simulink model "mcb_pmsm_foc_f28379d_dyno"  (R2024b)
settings: Solver=FixedStepDiscrete  StartTime=0.0  StopTime=10  RelTol=1e-3  EnableMultiTasking=on
InitFcn:
  | mcb_pmsm_foc_dyno_f28379d_data;
model workspace (MAT data in the model file):
  encoderResolution = 2000
  hallOffset = '0.5'
  indexOffset = 850
  polePairs = '4'
values from neighbouring files (symbols this model uses):
  dataType = 'single'    [mcb_pmsm_foc_dyno_f28379d_data.m]
  inverter_motor1 = mcb_updateInverterParameters(pmsm_motor1,inverter_motor1,target)    [mcb_pmsm_foc_dyno_f28379d_data.m]
  inverter_motor2 = mcb_updateInverterParameters(pmsm_motor2,inverter_motor2,target)    [mcb_pmsm_foc_dyno_f28379d_data.m]
  PI_params_motor1 = calculate_PI_params(pmsm_motor1,inverter_motor1)    [mcb_pmsm_foc_dyno_f28379d_data.m]
  PI_params_motor2 = calculate_PI_params(pmsm_motor2,inverter_motor2)    [mcb_pmsm_foc_dyno_f28379d_data.m]
  pmsm_motor1 = mcb_SetPMSMMotorParameters('Teknic2310P')    [mcb_pmsm_foc_dyno_f28379d_data.m]
  pmsm_motor2 = mcb_SetPMSMMotorParameters('Teknic2310P')    [mcb_pmsm_foc_dyno_f28379d_data.m]
  PU_System_motor1 = mcb_SetPUSystem(pmsm_motor1,inverter_motor1)    [mcb_pmsm_foc_dyno_f28379d_data.m]
  PU_System_motor2 = mcb_SetPUSystem(pmsm_motor2,inverter_motor2)    [mcb_pmsm_foc_dyno_f28379d_data.m]
  T_pwm = 1/PWM_frequency    (= 5e-05)    [mcb_pmsm_foc_dyno_f28379d_data.m]
  target = mcb_SetProcessorDetails('F28379D',PWM_frequency)    [mcb_pmsm_foc_dyno_f28379d_data.m]
  Ts = T_pwm    (= 5e-05)    [mcb_pmsm_foc_dyno_f28379d_data.m]
  Ts_inverter = T_pwm/2    (= 2.5e-05)    [mcb_pmsm_foc_dyno_f28379d_data.m]
  Ts_motor = T_pwm/2    (= 2.5e-05)    [mcb_pmsm_foc_dyno_f28379d_data.m]
  Ts_speed = 10*Ts    (= 0.0005)    [mcb_pmsm_foc_dyno_f28379d_data.m]
undefined symbols (not defined in the file or in its folder): DiscIntNeverNeededParam, Down, GPTRIP1SEL, GPTRIP2SEL, TZ1, TZ2, Up
libraries: mcbcontrolslib x22, c2802xlib x14, simulink x10, c2837xDlib x7, mcbpositiondecoderlib x6, slpidlib x5, c280xlib x5, mcbpmsmnonlinearlib x4, svdschedulerlib x3, autolibpmsmexterior x2, mcbplantlib x2, svdutilitieslib x1
(part 4 of 4)

== system mcb_pmsm_foc_f28379d_dyno/Current control for motor1/Control_System/Closed Loop Control/Current_Controllers/PI_Controller_Iq ==
  I_ref : Inport
  I_fb : Inport  Port=2
  Constant : Constant
  Data Store Read1 : DataStoreRead  DataStoreName=EnMtrCtrl  IndexOptions=Index vector (dialog)  Indices=1  OutputSizes=1
  Discrete PI Controller with anti-windup & reset : slpidlib/PID Controller  Controller=PI  Form=Parallel  TimeDomain=Discrete-time  UseExternalTs=off  SampleTime=-1  IntegratorMethod=Forward Euler  FilterMethod=Forward Euler  ControllerParametersSource=external  P=1  I=1  UseKiTs=on  D=0  UseExternalDerivativeSource=off  N=100  UseFilter=on  TunerSelectOption=Transfer Function Based (PID Tuner App)  InitialConditionSource=external  InitialConditionForIntegrator=0  InitialConditionForFilter=0  DifferentiatorICPrevScaledInput=0  ExternalReset=level  TrackingMode=off  Kt=1  LimitOutput=on  SatLimitsSource=internal  UpperSaturationLimit=1  LowerSaturationLimit=-1  LinearizeAsGain=on  AntiWindupMode=clamping  Kb=1  LimitIntegrator=off  UpperIntegratorSaturationLimit=inf  LowerIntegratorSaturationLimit=-inf  RndMeth=Simplest  POutMin=[]  POutMax=[]  IOutMin=[]  IOutMax=[]  DOutMin=[]  DOutMax=[]  NOutMin=[]  NOutMax=[]  SumOutMin=[]  SumOutMax=[]  SaturationOutDataTypeStr=Inherit: Inherit via back propagation  SaturationOutMin=[]  SaturationOutMax=[]  PParamMin=[]  PParamMax=[]  IParamMin=[]  IParamMax=[]  DParamMin=[]  DParamMax=[]  NParamMin=[]  NParamMax=[]  KbParamMin=[]  KbParamMax=[]  KtParamMin=[]  KtParamMax=[]  KbOutMin=[]  KbOutMax=[]  KtOutMin=[]  KtOutMax=[]  IntegratorOutMin=[]  IntegratorOutMax=[]  FilterOutMin=[]  FilterOutMax=[]  SumI1OutMin=[]  SumI1OutMax=[]  SumI2OutMin=[]  SumI2OutMax=[]  SumI3OutMin=[]  SumI3OutMax=[]  SumI4OutMin=[]  SumI4OutMax=[]  SumDOutMin=[]  SumDOutMax=[]  DifferentiatorOutMin=[]  DifferentiatorOutMax=[]  FilterDiffOutCoefMin=[]  FilterDiffOutCoefMax=[]  ReciprocalOutMin=[]  ReciprocalOutMax=[]  SumDenOutMin=[]  SumDenOutMax=[]  SumNumOutMin=[]  SumNumOutMax=[]  DivideOutMin=[]  DivideOutMax=[]  UdiffTsProdOutMin=[]  UdiffTsProdOutMax=[]  NTsProdOutMin=[]  NTsProdOutMax=[]  UintegralTsProdOutMin=[]  UintegralTsProdOutMax=[]  UngainTsProdOutMin=[]  UngainTsProdOutMax=[]  ClampingZeroOutDataTypeStr=Inherit: Inherit via back propagation  ClampingZeroOutMin=[]  ClampingZeroOutMax=[]  FilterDenConstantOutDataTypeStr=Inherit: Inherit via back propagation  FilterDenConstantOutMin=[]  FilterDenConstantOutMax=[]  PCopyOutDataTypeStr=Inherit: Inherit via back propagation  PCopyOutMin=[]  PCopyOutMax=[]  NCopyOutDataTypeStr=Inherit: Inherit via back propagation  NCopyOutMin=[]  NCopyOutMax=[]  IntegratorContinuousStateAttributes=''  IntegratorStateMustResolveToSignalObject=off  IntegratorRTWStateStorageClass=Auto  FilterContinuousStateAttributes=''  FilterStateMustResolveToSignalObject=off  FilterRTWStateStorageClass=Auto  ParallelPVariant=ExternalParameters  IdealPVariant=Disabled  IVariant=ExternalParameters  DVariant=Disabled  IntegratorVariant=Discrete  SatVariant=Enabled  AWVariant=DiscClampingParallel  PCopyVariant=Disabled  TRVariant=Disabled  FdbkBlocksVariant=Forward  IdealPFdbkVariant=Disabled  SatFdbkVariant=Disabled  DerivativeFilterVariant=Disabled  NVariant=Disabled  NCopyVariant=Disabled_SignalSpec  FilterICVariant=Disabled  IntegratorICVariant=ExternalICs  ExternalResetVariant=ExternalReset  TRSumVariant=Passthrough  SumFdbkVariant=Disabled  SumVariant=Sum_PI  TsampFilterVariant=InternalTs  TsampNgainVariant=Passthrough  TsampIntegralVariant=Disabled_SignalSpec  ExternalSaturationOutDataTypeStr=Inherit: Same as second input  DerivativeSourceVariant=Disabled  PreIntVariant=InternalPreInt
  Ki : Constant  Value=PI_params_motor1.Ki_i*Ts  OutDataTypeStr=dataType  SampleTime=-1
  Kp : Constant  Value=PI_params_motor1.Kp_i  OutDataTypeStr=dataType  SampleTime=-1
  Kp1 : Constant  Value=0  OutDataTypeStr=dataType  SampleTime=-1
  Logical Operator : Logic  Operator=NOT  IconShape=distinctive  AllPortsSameDT=off  OutDataTypeStr=boolean
  MATLAB Function : MATLAB Function  TreatAsAtomicUnit=on
  Sum : Sum  Inputs=|+-  OutDataTypeStr=Inherit: Same as first input
  V_ref : Outport  VectorParamsAs1DForOutWhenUnconnected=off
  wires:
  MATLAB Function/1(V_q_ref) -> V_ref/1
  Data Store Read1/1 -> Logical Operator/1
  I_fb/1 -> Sum/2
  I_ref/1 -> Sum/1
  Kp/1 -> MATLAB Function/2(P)
  Sum/1 -> MATLAB Function/1(e)
  Ki/1 -> MATLAB Function/3(I_Ts_speed)
  Logical Operator/1 -> MATLAB Function/4(reset)
  Kp1/1 -> MATLAB Function/5(Iq0)
  Constant/1 -> MATLAB Function/6(saturation_limit)

== system mcb_pmsm_foc_f28379d_dyno/Current control for motor1/Input Scaling/Calculate Phase Currents/Data_Type/Data_Type_Fixed_Point ==
  In1 : Inport
  Data Type Conversion : DataTypeConversion  OutDataTypeStr=fixdt(1,32,17)  ConvertRealWorld=Stored Integer (SI)  RndMeth=Simplest  SaturateOnIntegerOverflow=off
  Data Type Conversion1 : DataTypeConversion  OutDataTypeStr=dataType  RndMeth=Simplest  SaturateOnIntegerOverflow=off
  Q17 per unit conversion : ArithShift  BitShiftNumber=-6
  Iab_meas_PU : Outport
  wires:
  In1/1 -> Q17 per unit conversion/1
  Data Type Conversion1/1 -> Iab_meas_PU/1
  Data Type Conversion/1 -> Data Type Conversion1/1
  Q17 per unit conversion/1 -> Data Type Conversion/1

== system mcb_pmsm_foc_f28379d_dyno/Current control for motor1/Input Scaling/Calculate Phase Currents/Data_Type/Data_Type_Float ==
  In1 : Inport
  Get ADC Voltage : Gain  Gain=target.ADC_Vref /target.ADC_MaxCount  OutDataTypeStr=dataType  RndMeth=Simplest
  Get Currents : Gain  Gain=1/inverter_motor1.ISenseVoltPerAmp  RndMeth=Simplest  OutDataTypeStr=Inherit: Same as input
  PU_Conversion : Gain  Gain=1/PU_System_motor1.I_base  RndMeth=Simplest  OutDataTypeStr=Inherit: Same as input
  Iab_meas_PU : Outport
  wires:
  Get ADC Voltage/1 -> Get Currents/1
  Get Currents/1 -> PU_Conversion/1
  PU_Conversion/1 -> Iab_meas_PU/1
  In1/1 -> Get ADC Voltage/1

== system mcb_pmsm_foc_f28379d_dyno/Current control for motor1/SCI_Tx/Code Generation/Data_Conditioning_Tx/Data_Type_Fixed_Point ==
  In1 : Inport
  Data Type Conversion : DataTypeConversion  OutDataTypeStr=fixdt(1,32,28)  RndMeth=Simplest  SaturateOnIntegerOverflow=off
  Data Type Conversion3 : DataTypeConversion  OutDataTypeStr=uint32  ConvertRealWorld=Stored Integer (SI)  RndMeth=Simplest  SaturateOnIntegerOverflow=off
  Data_Log : Outport
  wires:
  In1/1 -> Data Type Conversion/1
  Data Type Conversion3/1 -> Data_Log/1
  Data Type Conversion/1 -> Data Type Conversion3/1

== system mcb_pmsm_foc_f28379d_dyno/Current control for motor1/SCI_Tx/Code Generation/Data_Conditioning_Tx/Data_Type_Float ==
  In1 : Inport
  Byte Pack : svdutilitieslib/Byte Pack  maskPackedDataType=uint32  datatypes={'single'}  byteAlign=4  blockPlatform=tic2000
  Data_Log : Outport
  wires:
  Byte Pack/1 -> Data_Log/1
  In1/1 -> Byte Pack/1

== system mcb_pmsm_foc_f28379d_dyno/Current control for motor1/SCI_Tx/Code Generation/Data_Logging/Data ==
  Data : Inport
  Data_width : Inport  Port=2
  Action Port : ActionPort  ActionPortLabel=else
  Dummy : Constant  Value=hex2dec('0000')  OutDataTypeStr=uint32
  Mux : Mux  Inputs=2
  Data_out : Outport  VectorParamsAs1DForOutWhenUnconnected=off
  Iteration : Outport  Port=2  VectorParamsAs1DForOutWhenUnconnected=off
  wires:
  Data_width/1 -> Iteration/1
  Data/1 -> Mux/1
  Dummy/1 -> Mux/2
  Mux/1 -> Data_out/1

== system mcb_pmsm_foc_f28379d_dyno/Current control for motor1/SCI_Tx/Code Generation/Data_Logging/End ==
  Data : Inport
  Data_width : Inport  Port=2
  Action Port : ActionPort  ActionPortLabel=elseif(u1 == 599)
  Bias : Bias  Bias=1  SaturateOnIntegerOverflow=off
  End : Constant  Value=hex2dec('45454545')  OutDataTypeStr=uint32
  Mux : Mux  Inputs=2
  Data_out : Outport  VectorParamsAs1DForOutWhenUnconnected=off
  Iteration : Outport  Port=2  VectorParamsAs1DForOutWhenUnconnected=off
  wires:
  Data/1 -> Mux/1
  Data_width/1 -> Bias/1
  Bias/1 -> Iteration/1
  End/1 -> Mux/2
  Mux/1 -> Data_out/1

== system mcb_pmsm_foc_f28379d_dyno/Current control for motor1/SCI_Tx/Code Generation/Data_Logging/Start ==
  Data : Inport
  Data_width : Inport  Port=2
  Action Port : ActionPort  ActionPortLabel=if(u1 == 0)
  Bias : Bias  Bias=1  SaturateOnIntegerOverflow=off
  Mux : Mux  Inputs=2
  Start : Constant  Value=hex2dec('53535353')  OutDataTypeStr=uint32
  Data_out : Outport  VectorParamsAs1DForOutWhenUnconnected=off
  Iteration : Outport  Port=2  VectorParamsAs1DForOutWhenUnconnected=off
  wires:
  Data/1 -> Mux/2
  Data_width/1 -> Bias/1
  Bias/1 -> Iteration/1
  Start/1 -> Mux/1
  Mux/1 -> Data_out/1

== system mcb_pmsm_foc_f28379d_dyno/Current control for motor2/Control_System/Closed Loop Control/Current_Controllers/PI_Controller_Id ==
  I_ref : Inport
  I_fb : Inport  Port=2
  Constant : Constant
  Data Store Read1 : DataStoreRead  DataStoreName=EnMtr2TrqCtrl  IndexOptions=Index vector (dialog)  Indices=1  OutputSizes=1
  Discrete PI Controller with anti-windup & reset : slpidlib/PID Controller  Controller=PI  Form=Parallel  TimeDomain=Discrete-time  UseExternalTs=off  SampleTime=-1  IntegratorMethod=Forward Euler  FilterMethod=Forward Euler  ControllerParametersSource=external  P=1  I=1  UseKiTs=on  D=0  UseExternalDerivativeSource=off  N=100  UseFilter=on  TunerSelectOption=Transfer Function Based (PID Tuner App)  InitialConditionSource=external  InitialConditionForIntegrator=0  InitialConditionForFilter=0  DifferentiatorICPrevScaledInput=0  ExternalReset=level  TrackingMode=off  Kt=1  LimitOutput=on  SatLimitsSource=internal  UpperSaturationLimit=1  LowerSaturationLimit=-1  LinearizeAsGain=on  AntiWindupMode=clamping  Kb=1  LimitIntegrator=off  UpperIntegratorSaturationLimit=inf  LowerIntegratorSaturationLimit=-inf  RndMeth=Simplest  POutMin=[]  POutMax=[]  IOutMin=[]  IOutMax=[]  DOutMin=[]  DOutMax=[]  NOutMin=[]  NOutMax=[]  SumOutMin=[]  SumOutMax=[]  SaturationOutDataTypeStr=Inherit: Inherit via back propagation  SaturationOutMin=[]  SaturationOutMax=[]  PParamMin=[]  PParamMax=[]  IParamMin=[]  IParamMax=[]  DParamMin=[]  DParamMax=[]  NParamMin=[]  NParamMax=[]  KbParamMin=[]  KbParamMax=[]  KtParamMin=[]  KtParamMax=[]  KbOutMin=[]  KbOutMax=[]  KtOutMin=[]  KtOutMax=[]  IntegratorOutMin=[]  IntegratorOutMax=[]  FilterOutMin=[]  FilterOutMax=[]  SumI1OutMin=[]  SumI1OutMax=[]  SumI2OutMin=[]  SumI2OutMax=[]  SumI3OutMin=[]  SumI3OutMax=[]  SumI4OutMin=[]  SumI4OutMax=[]  SumDOutMin=[]  SumDOutMax=[]  DifferentiatorOutMin=[]  DifferentiatorOutMax=[]  FilterDiffOutCoefMin=[]  FilterDiffOutCoefMax=[]  ReciprocalOutMin=[]  ReciprocalOutMax=[]  SumDenOutMin=[]  SumDenOutMax=[]  SumNumOutMin=[]  SumNumOutMax=[]  DivideOutMin=[]  DivideOutMax=[]  UdiffTsProdOutMin=[]  UdiffTsProdOutMax=[]  NTsProdOutMin=[]  NTsProdOutMax=[]  UintegralTsProdOutMin=[]  UintegralTsProdOutMax=[]  UngainTsProdOutMin=[]  UngainTsProdOutMax=[]  ClampingZeroOutDataTypeStr=Inherit: Inherit via back propagation  ClampingZeroOutMin=[]  ClampingZeroOutMax=[]  FilterDenConstantOutDataTypeStr=Inherit: Inherit via back propagation  FilterDenConstantOutMin=[]  FilterDenConstantOutMax=[]  PCopyOutDataTypeStr=Inherit: Inherit via back propagation  PCopyOutMin=[]  PCopyOutMax=[]  NCopyOutDataTypeStr=Inherit: Inherit via back propagation  NCopyOutMin=[]  NCopyOutMax=[]  IntegratorContinuousStateAttributes=''  IntegratorStateMustResolveToSignalObject=off  IntegratorRTWStateStorageClass=Auto  FilterContinuousStateAttributes=''  FilterStateMustResolveToSignalObject=off  FilterRTWStateStorageClass=Auto  ParallelPVariant=ExternalParameters  IdealPVariant=Disabled  IVariant=ExternalParameters  DVariant=Disabled  IntegratorVariant=Discrete  SatVariant=Enabled  AWVariant=DiscClampingParallel  PCopyVariant=Disabled  TRVariant=Disabled  FdbkBlocksVariant=Forward  IdealPFdbkVariant=Disabled  SatFdbkVariant=Disabled  DerivativeFilterVariant=Disabled  NVariant=Disabled  NCopyVariant=Disabled_SignalSpec  FilterICVariant=Disabled  IntegratorICVariant=ExternalICs  ExternalResetVariant=ExternalReset  TRSumVariant=Passthrough  SumFdbkVariant=Disabled  SumVariant=Sum_PI  TsampFilterVariant=InternalTs  TsampNgainVariant=Passthrough  TsampIntegralVariant=Disabled_SignalSpec  ExternalSaturationOutDataTypeStr=Inherit: Same as second input  DerivativeSourceVariant=Disabled  PreIntVariant=InternalPreInt
  Ki : Constant  Value=PI_params_motor2.Ki_i*Ts  OutDataTypeStr=dataType  SampleTime=-1
  Ki1 : Constant  Value=0  OutDataTypeStr=dataType  SampleTime=-1
  Kp : Constant  Value=PI_params_motor2.Kp_i  OutDataTypeStr=dataType  SampleTime=-1
  Logical Operator : Logic  Operator=NOT  IconShape=distinctive  AllPortsSameDT=off  OutDataTypeStr=boolean
  MATLAB Function : MATLAB Function  TreatAsAtomicUnit=on
  Sum : Sum  Inputs=|+-  OutDataTypeStr=Inherit: Same as first input
  V_ref : Outport  VectorParamsAs1DForOutWhenUnconnected=off
  wires:
  Ki1/1 -> MATLAB Function/5(Id0)
  Logical Operator/1 -> MATLAB Function/4(reset)
  Ki/1 -> MATLAB Function/3(I_Ts_speed)
  Kp/1 -> MATLAB Function/2(P)
  Sum/1 -> MATLAB Function/1(e)
  MATLAB Function/1(V_d_ref) -> V_ref/1
  Data Store Read1/1 -> Logical Operator/1
  I_fb/1 -> Sum/2
  I_ref/1 -> Sum/1
  Constant/1 -> MATLAB Function/6(saturation_limit)

== system mcb_pmsm_foc_f28379d_dyno/Current control for motor2/Control_System/Closed Loop Control/Current_Controllers/PI_Controller_Iq ==
  I_ref : Inport
  I_fb : Inport  Port=2
  Constant : Constant
  Data Store Read1 : DataStoreRead  DataStoreName=EnMtr2TrqCtrl  IndexOptions=Index vector (dialog)  Indices=1  OutputSizes=1
  Discrete PI Controller with anti-windup & reset : slpidlib/PID Controller  Controller=PI  Form=Parallel  TimeDomain=Discrete-time  UseExternalTs=off  SampleTime=-1  IntegratorMethod=Forward Euler  FilterMethod=Forward Euler  ControllerParametersSource=external  P=1  I=1  UseKiTs=on  D=0  UseExternalDerivativeSource=off  N=100  UseFilter=on  TunerSelectOption=Transfer Function Based (PID Tuner App)  InitialConditionSource=external  InitialConditionForIntegrator=0  InitialConditionForFilter=0  DifferentiatorICPrevScaledInput=0  ExternalReset=level  TrackingMode=off  Kt=1  LimitOutput=on  SatLimitsSource=internal  UpperSaturationLimit=1  LowerSaturationLimit=-1  LinearizeAsGain=on  AntiWindupMode=clamping  Kb=1  LimitIntegrator=off  UpperIntegratorSaturationLimit=inf  LowerIntegratorSaturationLimit=-inf  RndMeth=Simplest  POutMin=[]  POutMax=[]  IOutMin=[]  IOutMax=[]  DOutMin=[]  DOutMax=[]  NOutMin=[]  NOutMax=[]  SumOutMin=[]  SumOutMax=[]  SaturationOutDataTypeStr=Inherit: Inherit via back propagation  SaturationOutMin=[]  SaturationOutMax=[]  PParamMin=[]  PParamMax=[]  IParamMin=[]  IParamMax=[]  DParamMin=[]  DParamMax=[]  NParamMin=[]  NParamMax=[]  KbParamMin=[]  KbParamMax=[]  KtParamMin=[]  KtParamMax=[]  KbOutMin=[]  KbOutMax=[]  KtOutMin=[]  KtOutMax=[]  IntegratorOutMin=[]  IntegratorOutMax=[]  FilterOutMin=[]  FilterOutMax=[]  SumI1OutMin=[]  SumI1OutMax=[]  SumI2OutMin=[]  SumI2OutMax=[]  SumI3OutMin=[]  SumI3OutMax=[]  SumI4OutMin=[]  SumI4OutMax=[]  SumDOutMin=[]  SumDOutMax=[]  DifferentiatorOutMin=[]  DifferentiatorOutMax=[]  FilterDiffOutCoefMin=[]  FilterDiffOutCoefMax=[]  ReciprocalOutMin=[]  ReciprocalOutMax=[]  SumDenOutMin=[]  SumDenOutMax=[]  SumNumOutMin=[]  SumNumOutMax=[]  DivideOutMin=[]  DivideOutMax=[]  UdiffTsProdOutMin=[]  UdiffTsProdOutMax=[]  NTsProdOutMin=[]  NTsProdOutMax=[]  UintegralTsProdOutMin=[]  UintegralTsProdOutMax=[]  UngainTsProdOutMin=[]  UngainTsProdOutMax=[]  ClampingZeroOutDataTypeStr=Inherit: Inherit via back propagation  ClampingZeroOutMin=[]  ClampingZeroOutMax=[]  FilterDenConstantOutDataTypeStr=Inherit: Inherit via back propagation  FilterDenConstantOutMin=[]  FilterDenConstantOutMax=[]  PCopyOutDataTypeStr=Inherit: Inherit via back propagation  PCopyOutMin=[]  PCopyOutMax=[]  NCopyOutDataTypeStr=Inherit: Inherit via back propagation  NCopyOutMin=[]  NCopyOutMax=[]  IntegratorContinuousStateAttributes=''  IntegratorStateMustResolveToSignalObject=off  IntegratorRTWStateStorageClass=Auto  FilterContinuousStateAttributes=''  FilterStateMustResolveToSignalObject=off  FilterRTWStateStorageClass=Auto  ParallelPVariant=ExternalParameters  IdealPVariant=Disabled  IVariant=ExternalParameters  DVariant=Disabled  IntegratorVariant=Discrete  SatVariant=Enabled  AWVariant=DiscClampingParallel  PCopyVariant=Disabled  TRVariant=Disabled  FdbkBlocksVariant=Forward  IdealPFdbkVariant=Disabled  SatFdbkVariant=Disabled  DerivativeFilterVariant=Disabled  NVariant=Disabled  NCopyVariant=Disabled_SignalSpec  FilterICVariant=Disabled  IntegratorICVariant=ExternalICs  ExternalResetVariant=ExternalReset  TRSumVariant=Passthrough  SumFdbkVariant=Disabled  SumVariant=Sum_PI  TsampFilterVariant=InternalTs  TsampNgainVariant=Passthrough  TsampIntegralVariant=Disabled_SignalSpec  ExternalSaturationOutDataTypeStr=Inherit: Same as second input  DerivativeSourceVariant=Disabled  PreIntVariant=InternalPreInt
  Ki : Constant  Value=PI_params_motor2.Ki_i*Ts  OutDataTypeStr=dataType  SampleTime=-1
  Kp : Constant  Value=PI_params_motor2.Kp_i  OutDataTypeStr=dataType  SampleTime=-1
  Kp1 : Constant  Value=0  OutDataTypeStr=dataType  SampleTime=-1
  Logical Operator : Logic  Operator=NOT  IconShape=distinctive  AllPortsSameDT=off  OutDataTypeStr=boolean
  MATLAB Function : MATLAB Function  TreatAsAtomicUnit=on
  Sum : Sum  Inputs=|+-  OutDataTypeStr=Inherit: Same as first input
  V_ref : Outport  VectorParamsAs1DForOutWhenUnconnected=off
  wires:
  Kp1/1 -> MATLAB Function/5(Iq0)
  Logical Operator/1 -> MATLAB Function/4(reset)
  Ki/1 -> MATLAB Function/3(I_Ts_speed)
  Sum/1 -> MATLAB Function/1(e)
  Kp/1 -> MATLAB Function/2(P)
  I_ref/1 -> Sum/1
  I_fb/1 -> Sum/2
  Data Store Read1/1 -> Logical Operator/1
  MATLAB Function/1(V_q_ref) -> V_ref/1
  Constant/1 -> MATLAB Function/6(saturation_limit)

== system mcb_pmsm_foc_f28379d_dyno/Current control for motor2/Enable Motor2 after a delay/Delay to start motor1 (codegen)/Enable EnMtr2TrqCtrl after 2 sec delay/Enable EnMtr2TrqCtrl ==
  Enable : EnablePort  StatesWhenEnabling=reset
  Constant : Constant  OutDataTypeStr=boolean
  Data Store Write : DataStoreWrite  DataStoreName=EnMtr2TrqCtrl  IndexOptions=Index vector (dialog)  Indices=1  OutputSizes=1
  GPIO Trig : Constant  OutDataTypeStr=uint16  SampleTime=-1
  GPIO16 : c2837xDlib/Digital Output  GPIO_Number=GPIO16~GPIO23  GPIO_Bit0=on  GPIO_BIT0_Toggle=off  GPIO_Bit1=off  GPIO_BIT1_Toggle=off  GPIO_Bit2=off  GPIO_BIT2_Toggle=off  GPIO_Bit3=off  GPIO_BIT3_Toggle=off  GPIO_Bit4=off  GPIO_BIT4_Toggle=off  GPIO_Bit5=off  GPIO_BIT5_Toggle=off  GPIO_Bit6=off  GPIO_BIT6_Toggle=off  GPIO_Bit7=off  GPIO_BIT7_Toggle=off
  wires:
  Constant/1 -> Data Store Write/1
  GPIO Trig/1 -> GPIO16/1

== system mcb_pmsm_foc_f28379d_dyno/Current control for motor2/Input Scaling/Calculate Phase Currents/Data_Type/Data_Type_Fixed_Point ==
  In1 : Inport
  Data Type Conversion : DataTypeConversion  OutDataTypeStr=fixdt(1,32,17)  ConvertRealWorld=Stored Integer (SI)  RndMeth=Simplest  SaturateOnIntegerOverflow=off
  Data Type Conversion1 : DataTypeConversion  OutDataTypeStr=dataType  RndMeth=Simplest  SaturateOnIntegerOverflow=off
  Q17 per unit conversion : ArithShift  BitShiftNumber=-6
  Iab_meas_PU : Outport
  wires:
  Q17 per unit conversion/1 -> Data Type Conversion/1
  Data Type Conversion/1 -> Data Type Conversion1/1
  Data Type Conversion1/1 -> Iab_meas_PU/1
  In1/1 -> Q17 per unit conversion/1

== system mcb_pmsm_foc_f28379d_dyno/Current control for motor2/Input Scaling/Calculate Phase Currents/Data_Type/Data_Type_Float ==
  In1 : Inport
  Get ADC Voltage : Gain  Gain=target.ADC_Vref /target.ADC_MaxCount  OutDataTypeStr=dataType  RndMeth=Simplest
  Get Currents : Gain  Gain=1/inverter_motor2.ISenseVoltPerAmp  RndMeth=Simplest  OutDataTypeStr=Inherit: Same as input
  PU_Conversion : Gain  Gain=1/PU_System_motor2.I_base  RndMeth=Simplest  OutDataTypeStr=Inherit: Same as input
  Iab_meas_PU : Outport
  wires:
  Get ADC Voltage/1 -> Get Currents/1
  Get Currents/1 -> PU_Conversion/1
  PU_Conversion/1 -> Iab_meas_PU/1
  In1/1 -> Get ADC Voltage/1

== system mcb_pmsm_foc_f28379d_dyno/Hardware Init/HW_Init/HW_Init (Codegen)/Calibrate ADC offset for motor 1 current sensor/Calculate ADC Offset  ==
  Enable : EnablePort
  Constant : Constant  Value=8
  Constant1 : Constant  Value=inverter_motor1.CtSensOffsetMax  OutDataTypeStr=Inherit: Inherit via back propagation
  Constant2 : Constant  Value=inverter_motor1.CtSensOffsetMin  OutDataTypeStr=Inherit: Inherit via back propagation
  Divide : Product  Inputs=*/  OutDataTypeStr=uint16
  Divide1 : Product  Inputs=*/  OutDataTypeStr=uint16
  For Iterator Subsystem : Subsystem  TreatAsAtomicUnit=on
  If : If  NumInputs=3  IfExpression=u1 > u3 & u1 < u2
  If Action Subsystem : Subsystem  TreatAsAtomicUnit=on
  If Action Subsystem1 : Subsystem  TreatAsAtomicUnit=on
  If Action Subsystem2 : Subsystem  TreatAsAtomicUnit=on
  If Action Subsystem3 : Subsystem  TreatAsAtomicUnit=on
  If1 : If  NumInputs=3  IfExpression=u1 > u3 & u1 < u2
  wires:
  For Iterator Subsystem/2(Out2) -> Divide1/1
  Divide/1 -> If Action Subsystem/1(In1), If/1
  For Iterator Subsystem/1(Out1) -> Divide/1
  Constant/1 -> Divide/2, Divide1/2
  Divide1/1 -> If1/1, If Action Subsystem2/1(In1)
  If/1 -> If Action Subsystem/Action
  If/2 -> If Action Subsystem1/Action
  If1/1 -> If Action Subsystem2/Action
  If1/2 -> If Action Subsystem3/Action
  Constant1/1 -> If/2, If1/2
  Constant2/1 -> If/3, If1/3

== system mcb_pmsm_foc_f28379d_dyno/Hardware Init/HW_Init/HW_Init (Codegen)/Calibrate ADC offset for motor 1 current sensor/Default ADC Offset ==
  Enable : EnablePort
  Constant : Constant  Value=inverter_motor1.CtSensAOffset  OutDataTypeStr=Inherit: Inherit via back propagation
  Constant1 : Constant  Value=inverter_motor1.CtSensBOffset  OutDataTypeStr=Inherit: Inherit via back propagation
  Data Store Write1 : DataStoreWrite  DataStoreName=IaOffset_motor1  IndexOptions=Index vector (dialog)  Indices=1  OutputSizes=1
  Data Store Write2 : DataStoreWrite  DataStoreName=IbOffset_motor1  IndexOptions=Index vector (dialog)  Indices=1  OutputSizes=1
  wires:
  Constant/1 -> Data Store Write1/1
  Constant1/1 -> Data Store Write2/1

== system mcb_pmsm_foc_f28379d_dyno/Hardware Init/HW_Init/HW_Init (Codegen)/Calibrate ADC offset for motor 2 current sensor/Calculate ADC Offset  ==
  Enable : EnablePort
  Constant1 : Constant  Value=8
  Constant2 : Constant  Value=inverter_motor2.CtSensOffsetMax  OutDataTypeStr=Inherit: Inherit via back propagation
  Constant3 : Constant  Value=inverter_motor2.CtSensOffsetMin  OutDataTypeStr=Inherit: Inherit via back propagation
  Divide2 : Product  Inputs=*/  OutDataTypeStr=uint16
  Divide3 : Product  Inputs=*/  OutDataTypeStr=uint16
  For Iterator Subsystem : Subsystem  TreatAsAtomicUnit=on
  If Action Subsystem4 : Subsystem  TreatAsAtomicUnit=on
  If Action Subsystem5 : Subsystem  TreatAsAtomicUnit=on
  If Action Subsystem6 : Subsystem  TreatAsAtomicUnit=on
  If Action Subsystem7 : Subsystem  TreatAsAtomicUnit=on
  If2 : If  NumInputs=3  IfExpression=u1 > u3 & u1 < u2
  If3 : If  NumInputs=3  IfExpression=u1 > u3 & u1 < u2
  wires:
  For Iterator Subsystem/2(Out4) -> Divide3/1
  Divide2/1 -> If2/1, If Action Subsystem4/1(In1)
  For Iterator Subsystem/1(Out3) -> Divide2/1
  Constant1/1 -> Divide2/2, Divide3/2
  Divide3/1 -> If3/1, If Action Subsystem6/1(In1)
  If2/1 -> If Action Subsystem4/Action
  If2/2 -> If Action Subsystem5/Action
  If3/1 -> If Action Subsystem6/Action
  If3/2 -> If Action Subsystem7/Action
  Constant2/1 -> If2/2, If3/2
  Constant3/1 -> If2/3, If3/3

== system mcb_pmsm_foc_f28379d_dyno/Hardware Init/HW_Init/HW_Init (Codegen)/Calibrate ADC offset for motor 2 current sensor/Default ADC Offset ==
  Enable : EnablePort
  Constant2 : Constant  Value=inverter_motor2.CtSensAOffset  OutDataTypeStr=Inherit: Inherit via back propagation
  Constant3 : Constant  Value=inverter_motor2.CtSensBOffset  OutDataTypeStr=Inherit: Inherit via back propagation
  Data Store Write3 : DataStoreWrite  DataStoreName=IaOffset_motor2  IndexOptions=Index vector (dialog)  Indices=1  OutputSizes=1
  Data Store Write4 : DataStoreWrite  DataStoreName=IbOffset_motor2  IndexOptions=Index vector (dialog)  Indices=1  OutputSizes=1
  wires:
  Constant2/1 -> Data Store Write3/1
  Constant3/1 -> Data Store Write4/1

== system mcb_pmsm_foc_f28379d_dyno/Serial Receive/SCI_Rx/Code generation/Serial Rx/Data_Type_Fixed_Point ==
  SCI Receive : c280xlib/SCI Receive  sciModule=A  dataHead=''  headerCheckMaxCount=16  dataTail=''  dataType=uint32  dataLenOptions=Length via dialog  dataDim=4  maxDataLength=1  initValue=0  errOption=Output the last received value  errValue=0  sampleTime=-1  blockingMode=on  timeOut=0.00875  outputStatus=off
  Rx : Outport
  wires:
  SCI Receive/1 -> Rx/1

== system mcb_pmsm_foc_f28379d_dyno/Serial Receive/SCI_Rx/Code generation/Serial Rx/Data_Type_Float ==
  SCI Receive : c280xlib/SCI Receive  sciModule=A  dataHead=''  headerCheckMaxCount=16  dataTail=''  dataType=single  dataLenOptions=Length via dialog  dataDim=4  maxDataLength=1  initValue=0  errOption=Output the last received value  errValue=0  sampleTime=-1  blockingMode=on  timeOut=0.00875  outputStatus=off
  Rx : Outport
  wires:
  SCI Receive/1 -> Rx/1

== system mcb_pmsm_foc_f28379d_dyno/Serial Receive/SCI_Rx/Simulation/Signal Packing/Data_Conditioning_Tx ==
  In1 : Inport
  In2 : Inport  Port=2
  In3 : Inport  Port=3
  In4 : Inport  Port=4
  Data_Type_Fixed_Point : Subsystem  VariantControl=~isequal(dataType, 'single')
  Data_Type_Float : Subsystem  VariantControl=isequal(dataType, 'single')
  Data : Outport

== system mcb_pmsm_foc_f28379d_dyno/Serial Receive/SCI_Rx/Simulation/Signal Packing/Parse ==
  Enable_PWM : Inport
  Debug_signals : Inport  Port=2
  Bitwise Operator : simulink/Logic and Bit Operations/Bitwise Operator  logicop=AND  UseBitMask=on  BitMask=hex2dec('0001')  BitMaskRealWorld=Stored Integer
  Bitwise Operator1 : simulink/Logic and Bit Operations/Bitwise Operator  logicop=AND  UseBitMask=on  BitMask=hex2dec('00F0')  BitMaskRealWorld=Stored Integer
  Shift Arithmetic1 : ArithShift  BitShiftNumber=-4
  Sum : Sum
  Data : Outport
  wires:
  Bitwise Operator/1 -> Sum/1
  Debug_signals/1 -> Shift Arithmetic1/1
  Sum/1 -> Data/1
  Shift Arithmetic1/1 -> Bitwise Operator1/1
  Enable_PWM/1 -> Bitwise Operator/1
  Bitwise Operator1/1 -> Sum/2

== system mcb_pmsm_foc_f28379d_dyno/Hardware Init/HW_Init/HW_Init (Codegen)/Calibrate ADC offset for motor 1 current sensor/Calculate ADC Offset /For Iterator Subsystem ==
  ADC_A_IN0 : c2802xlib/ADC  Priority=20  blkParamProc=C2000_Type4  ADCModule=C  samplingMode=Single sample mode  ADCResolution=12-bit (Single-ended input)  useSOC1=SOC2  useSOC2=SOC0_SOC1  SOCAcquisitionWindow=15  SOCTriggerSource=Software  SOCInterruptTrigger=No ADCINT  Ts=-1  dType=uint16  postInterrupt=off  interruptSel=ADCINT1  ADCINTContinuous=on  endma=off  chdma=1  conv1=ADCINA0  conv2=ADCINA0 and ADCINB0  conv1_Type4=ADCIN2  conv2_Type4=ADCIN0 and ADCIN1
  ADC_B_IN0 : c2802xlib/ADC  Priority=20  blkParamProc=C2000_Type4  ADCModule=B  samplingMode=Single sample mode  ADCResolution=12-bit (Single-ended input)  useSOC1=SOC2  useSOC2=SOC0_SOC1  SOCAcquisitionWindow=15  SOCTriggerSource=Software  SOCInterruptTrigger=No ADCINT  Ts=-1  dType=uint16  postInterrupt=off  interruptSel=ADCINT1  ADCINTContinuous=on  endma=off  chdma=1  conv1=ADCINA0  conv2=ADCINA0 and ADCINB0  conv1_Type4=ADCIN2  conv2_Type4=ADCIN0 and ADCIN1
  For Iterator : ForIterator  IterationLimit=16  IterationVariableDataType=uint16
  If : If  IfExpression=u1 > 8  ShowElse=off
  If Action Subsystem : Subsystem  TreatAsAtomicUnit=on
  Out1 : Outport
  Out2 : Outport  Port=2
  wires:
  For Iterator/1 -> If/1
  ADC_A_IN0/1 -> If Action Subsystem/1(In1)
  ADC_B_IN0/1 -> If Action Subsystem/2(In2)
  If Action Subsystem/1(Out1) -> Out1/1
  If Action Subsystem/2(Out2) -> Out2/1
  If/1 -> If Action Subsystem/Action

== system mcb_pmsm_foc_f28379d_dyno/Hardware Init/HW_Init/HW_Init (Codegen)/Calibrate ADC offset for motor 1 current sensor/Calculate ADC Offset /If Action Subsystem ==
  In1 : Inport
  Action Port : ActionPort  ActionPortLabel=if(u1 > u3 & u1 < u2)
  Data Store Write1 : DataStoreWrite  DataStoreName=IaOffset_motor1  IndexOptions=Index vector (dialog)  Indices=1  OutputSizes=1
  wires:
  In1/1 -> Data Store Write1/1

== system mcb_pmsm_foc_f28379d_dyno/Hardware Init/HW_Init/HW_Init (Codegen)/Calibrate ADC offset for motor 1 current sensor/Calculate ADC Offset /If Action Subsystem1 ==
  Action Port : ActionPort  ActionPortLabel=else
  Constant : Constant  Value=inverter_motor1.CtSensAOffset  OutDataTypeStr=Inherit: Inherit via back propagation
  Data Store Write1 : DataStoreWrite  DataStoreName=IaOffset_motor1  IndexOptions=Index vector (dialog)  Indices=1  OutputSizes=1
  wires:
  Constant/1 -> Data Store Write1/1

== system mcb_pmsm_foc_f28379d_dyno/Hardware Init/HW_Init/HW_Init (Codegen)/Calibrate ADC offset for motor 1 current sensor/Calculate ADC Offset /If Action Subsystem2 ==
  In1 : Inport
  Action Port : ActionPort  ActionPortLabel=if(u1 > u3 & u1 < u2)
  Data Store Write2 : DataStoreWrite  DataStoreName=IbOffset_motor1  IndexOptions=Index vector (dialog)  Indices=1  OutputSizes=1
  wires:
  In1/1 -> Data Store Write2/1

== system mcb_pmsm_foc_f28379d_dyno/Hardware Init/HW_Init/HW_Init (Codegen)/Calibrate ADC offset for motor 1 current sensor/Calculate ADC Offset /If Action Subsystem3 ==
  Action Port : ActionPort  ActionPortLabel=else
  Constant1 : Constant  Value=inverter_motor1.CtSensBOffset  OutDataTypeStr=Inherit: Inherit via back propagation
  Data Store Write2 : DataStoreWrite  DataStoreName=IbOffset_motor1  IndexOptions=Index vector (dialog)  Indices=1  OutputSizes=1
  wires:
  Constant1/1 -> Data Store Write2/1

== system mcb_pmsm_foc_f28379d_dyno/Hardware Init/HW_Init/HW_Init (Codegen)/Calibrate ADC offset for motor 2 current sensor/Calculate ADC Offset /For Iterator Subsystem ==
  ADC_A_IN1 : c2802xlib/ADC  Priority=20  blkParamProc=C2000_Type4  ADCModule=C  samplingMode=Single sample mode  ADCResolution=12-bit (Single-ended input)  useSOC1=SOC3  useSOC2=SOC0_SOC1  SOCAcquisitionWindow=15  SOCTriggerSource=Software  SOCInterruptTrigger=No ADCINT  Ts=-1  dType=uint16  postInterrupt=off  interruptSel=ADCINT1  ADCINTContinuous=on  endma=off  chdma=1  conv1=ADCINA0  conv2=ADCINA0 and ADCINB0  conv1_Type4=ADCIN4  conv2_Type4=ADCIN0 and ADCIN1
  ADC_B_IN1 : c2802xlib/ADC  Priority=20  blkParamProc=C2000_Type4  ADCModule=B  samplingMode=Single sample mode  ADCResolution=12-bit (Single-ended input)  useSOC1=SOC3  useSOC2=SOC0_SOC1  SOCAcquisitionWindow=15  SOCTriggerSource=Software  SOCInterruptTrigger=No ADCINT  Ts=-1  dType=uint16  postInterrupt=off  interruptSel=ADCINT1  ADCINTContinuous=on  endma=off  chdma=1  conv1=ADCINA0  conv2=ADCINA0 and ADCINB0  conv1_Type4=ADCIN4  conv2_Type4=ADCIN0 and ADCIN1
  For Iterator : ForIterator  IterationLimit=16  IterationVariableDataType=uint16
  If Action Subsystem1 : Subsystem  TreatAsAtomicUnit=on
  If1 : If  IfExpression=u1 > 8  ShowElse=off
  Out3 : Outport
  Out4 : Outport  Port=2
  wires:
  If1/1 -> If Action Subsystem1/Action
  If Action Subsystem1/2(Out2) -> Out4/1
  If Action Subsystem1/1(Out1) -> Out3/1
  ADC_B_IN1/1 -> If Action Subsystem1/2(In2)
  ADC_A_IN1/1 -> If Action Subsystem1/1(In1)
  For Iterator/1 -> If1/1

== system mcb_pmsm_foc_f28379d_dyno/Hardware Init/HW_Init/HW_Init (Codegen)/Calibrate ADC offset for motor 2 current sensor/Calculate ADC Offset /If Action Subsystem4 ==
  In1 : Inport
  Action Port : ActionPort  ActionPortLabel=if(u1 > u3 & u1 < u2)
  Data Store Write1 : DataStoreWrite  DataStoreName=IaOffset_motor2  IndexOptions=Index vector (dialog)  Indices=1  OutputSizes=1
  wires:
  In1/1 -> Data Store Write1/1

== system mcb_pmsm_foc_f28379d_dyno/Hardware Init/HW_Init/HW_Init (Codegen)/Calibrate ADC offset for motor 2 current sensor/Calculate ADC Offset /If Action Subsystem5 ==
  Action Port : ActionPort  ActionPortLabel=else
  Constant : Constant  Value=inverter_motor2.CtSensAOffset  OutDataTypeStr=Inherit: Inherit via back propagation
  Data Store Write1 : DataStoreWrite  DataStoreName=IaOffset_motor2  IndexOptions=Index vector (dialog)  Indices=1  OutputSizes=1
  wires:
  Constant/1 -> Data Store Write1/1

== system mcb_pmsm_foc_f28379d_dyno/Hardware Init/HW_Init/HW_Init (Codegen)/Calibrate ADC offset for motor 2 current sensor/Calculate ADC Offset /If Action Subsystem6 ==
  In1 : Inport
  Action Port : ActionPort  ActionPortLabel=if(u1 > u3 & u1 < u2)
  Data Store Write2 : DataStoreWrite  DataStoreName=IbOffset_motor2  IndexOptions=Index vector (dialog)  Indices=1  OutputSizes=1
  wires:
  In1/1 -> Data Store Write2/1

== system mcb_pmsm_foc_f28379d_dyno/Hardware Init/HW_Init/HW_Init (Codegen)/Calibrate ADC offset for motor 2 current sensor/Calculate ADC Offset /If Action Subsystem7 ==
  Action Port : ActionPort  ActionPortLabel=else
  Constant1 : Constant  Value=inverter_motor2.CtSensBOffset  OutDataTypeStr=Inherit: Inherit via back propagation
  Data Store Write2 : DataStoreWrite  DataStoreName=IbOffset_motor2  IndexOptions=Index vector (dialog)  Indices=1  OutputSizes=1
  wires:
  Constant1/1 -> Data Store Write2/1

== system mcb_pmsm_foc_f28379d_dyno/Serial Receive/SCI_Rx/Simulation/Signal Packing/Data_Conditioning_Tx/Data_Type_Fixed_Point ==
  In1 : Inport
  In2 : Inport  Port=2
  In3 : Inport  Port=3
  In4 : Inport  Port=4
  Data Type Conversion : DataTypeConversion  OutDataTypeStr=fixdt(1,32,28)  RndMeth=Simplest  SaturateOnIntegerOverflow=off
  Data Type Conversion1 : DataTypeConversion  OutDataTypeStr=uint32  RndMeth=Simplest  SaturateOnIntegerOverflow=off
  Data Type Conversion2 : DataTypeConversion  OutDataTypeStr=fixdt(1,32,28)  RndMeth=Simplest  SaturateOnIntegerOverflow=off
  Data Type Conversion3 : DataTypeConversion  OutDataTypeStr=uint32  ConvertRealWorld=Stored Integer (SI)  RndMeth=Simplest  SaturateOnIntegerOverflow=off
  Data Type Conversion4 : DataTypeConversion  OutDataTypeStr=uint32  ConvertRealWorld=Stored Integer (SI)  RndMeth=Simplest  SaturateOnIntegerOverflow=off
  Data Type Conversion5 : DataTypeConversion  OutDataTypeStr=fixdt(1,32,28)  RndMeth=Simplest  SaturateOnIntegerOverflow=off
  Data Type Conversion6 : DataTypeConversion  OutDataTypeStr=uint32  ConvertRealWorld=Stored Integer (SI)  RndMeth=Simplest  SaturateOnIntegerOverflow=off
  Mux : Mux
  Data : Outport
  wires:
  In1/1 -> Data Type Conversion/1
  Data Type Conversion3/1 -> Mux/1
  Data Type Conversion/1 -> Data Type Conversion3/1
  In2/1 -> Data Type Conversion1/1
  Data Type Conversion1/1 -> Mux/2
  Mux/1 -> Data/1
  Data Type Conversion2/1 -> Data Type Conversion4/1
  Data Type Conversion4/1 -> Mux/3
  In3/1 -> Data Type Conversion2/1
  Data Type Conversion5/1 -> Data Type Conversion6/1
  In4/1 -> Data Type Conversion5/1
  Data Type Conversion6/1 -> Mux/4

== system mcb_pmsm_foc_f28379d_dyno/Serial Receive/SCI_Rx/Simulation/Signal Packing/Data_Conditioning_Tx/Data_Type_Float ==
  In1 : Inport
  In2 : Inport  Port=2
  In3 : Inport  Port=3
  In4 : Inport  Port=4
  Data Type Conversion2 : DataTypeConversion  OutDataTypeStr=single  RndMeth=Simplest  SaturateOnIntegerOverflow=off
  Mux : Mux
  Data : Outport
  wires:
  In1/1 -> Mux/1
  Mux/1 -> Data/1
  In2/1 -> Data Type Conversion2/1
  Data Type Conversion2/1 -> Mux/2
  In3/1 -> Mux/3
  In4/1 -> Mux/4

== system mcb_pmsm_foc_f28379d_dyno/Hardware Init/HW_Init/HW_Init (Codegen)/Calibrate ADC offset for motor 1 current sensor/Calculate ADC Offset /For Iterator Subsystem/If Action Subsystem ==
  In1 : Inport
  In2 : Inport  Port=2
  Action Port : ActionPort  ActionPortLabel=if(u1 > 8)
  Memory : Memory  InheritSampleTime=on
  Memory1 : Memory  InheritSampleTime=on
  Sum : Sum
  Sum1 : Sum
  Out1 : Outport
  Out2 : Outport  Port=2
  wires:
  In1/1 -> Sum/1
  Sum/1 -> Out1/1, Memory/1
  In2/1 -> Sum1/1
  Memory/1 -> Sum/2
  Sum1/1 -> Out2/1, Memory1/1
  Memory1/1 -> Sum1/2

== system mcb_pmsm_foc_f28379d_dyno/Hardware Init/HW_Init/HW_Init (Codegen)/Calibrate ADC offset for motor 2 current sensor/Calculate ADC Offset /For Iterator Subsystem/If Action Subsystem1 ==
  In1 : Inport
  In2 : Inport  Port=2
  Action Port : ActionPort  ActionPortLabel=if(u1 > 8)
  Memory : Memory  InheritSampleTime=on
  Memory1 : Memory  InheritSampleTime=on
  Sum : Sum
  Sum1 : Sum
  Out1 : Outport
  Out2 : Outport  Port=2
  wires:
  In1/1 -> Sum/1
  Sum/1 -> Out1/1, Memory/1
  In2/1 -> Sum1/1
  Memory/1 -> Sum/2
  Sum1/1 -> Out2/1, Memory1/1
  Memory1/1 -> Sum1/2

== matlab function mcb_pmsm_foc_f28379d_dyno/Current control for motor1/Control_System/Closed Loop Control/Current_Controllers/PI_Controller_Id/MATLAB Function ==
  data: e input; V_d_ref output; P input; I_Ts_speed input; reset input; Id0 input; saturation_limit input
function V_d_ref = PI_Controller(e, P, I_Ts_speed, reset, Id0, saturation_limit)
    % PI_Controller: implementa un controllore PI con saturazione e reset.
    % INPUTS:
    % e               -> Errore (input del PI)
    % P               -> Guadagno proporzionale
    % I_Ts_speed      -> Guadagno integrale moltiplicato per Ts (I*Ts_speed)
    % reset           -> Segnale booleano per resettare l'integratore
    % Id0              -> Valore iniziale del riferimento (per l'integratore)
    % saturation_limit -> Limite di saturazione (valore assoluto)
    %
    % OUTPUT:
    % V_d_ref         -> Uscita del controllore PI con saturazione
    
    % Definizione di variabili statiche per la memoria interna del PI
    persistent integrator_state;
    if isempty(integrator_state)
        integrator_state = single(0);  % Inizializza la memoria dell'integratore
    end
    
    % Reset integratore se richiesto
    if reset
        integrator_state = Id0;
    end
    
    % Parte proporzionale
    P_term = P * e;
    
    % Parte integrale (accumulatore)
    integrator_state = integrator_state + I_Ts_speed * e;
    
    % Uscita PI senza saturazione
    V_d_ref_unsat = P_term + integrator_state;
    
    % Saturazione dell'uscita (limite superiore e inferiore)
    V_d_ref = max(min(V_d_ref_unsat, saturation_limit), -saturation_limit);
    
    % Implementazione dell'anti-windup: corregge l'integratore in caso di saturazione
    if V_d_ref ~= V_d_ref_unsat
        integrator_state = integrator_state - I_Ts_speed * e;  % Evita windup
    end
end

== matlab function mcb_pmsm_foc_f28379d_dyno/Speed control for motor1/PI_Controller_Speed/MATLAB Function ==
  data: e input; Trq_ref output; P input; I_Ts_speed input; reset input; I0 input; saturation_limit input
function Trq_ref = PI_Controller(e, P, I_Ts_speed, reset, I0, saturation_limit)
    % PI_Controller: implementa un controllore PI con saturazione e reset.
    % INPUTS:
    % e               -> Errore (input del PI)
    % P               -> Guadagno proporzionale
    % I_Ts_speed      -> Guadagno integrale moltiplicato per Ts (I*Ts_speed)
    % reset           -> Segnale booleano per resettare l'integratore
    % I0              -> Valore iniziale del riferimento (per l'integratore)
    % saturation_limit -> Limite di saturazione (valore assoluto)
    %
    % OUTPUT:
    % Trq_ref         -> Uscita del controllore PI con saturazione
    
    % Definizione di variabili statiche per la memoria interna del PI
    persistent integrator_state;
    if isempty(integrator_state)
        integrator_state = single(0);  % Inizializza la memoria dell'integratore
    end
    
    % Reset integratore se richiesto
    if reset
        integrator_state = I0;
    end
    
    % Parte proporzionale
    P_term = P * e;
    
    % Parte integrale (accumulatore)
    integrator_state = integrator_state + I_Ts_speed * e;
    
    % Uscita PI senza saturazione
    Trq_ref_unsat = P_term + integrator_state;
    
    % Saturazione dell'uscita (limite superiore e inferiore)
    Trq_ref = max(min(Trq_ref_unsat, saturation_limit), -saturation_limit);
    
    % Implementazione dell'anti-windup: corregge l'integratore in caso di saturazione
    if Trq_ref ~= Trq_ref_unsat
        integrator_state = integrator_state - I_Ts_speed * e;  % Evita windup
    end
end

== matlab function mcb_pmsm_foc_f28379d_dyno/Current control for motor2/Control_System/Closed Loop Control/Current_Controllers/PI_Controller_Id/MATLAB Function ==
  data: e input; V_d_ref output; P input; I_Ts_speed input; reset input; Id0 input; saturation_limit input
function V_d_ref = PI_Controller(e, P, I_Ts_speed, reset, Id0, saturation_limit)
    % PI_Controller: implementa un controllore PI con saturazione e reset.
    % INPUTS:
    % e               -> Errore (input del PI)
    % P               -> Guadagno proporzionale
    % I_Ts_speed      -> Guadagno integrale moltiplicato per Ts (I*Ts_speed)
    % reset           -> Segnale booleano per resettare l'integratore
    % Id0              -> Valore iniziale del riferimento (per l'integratore)
    % saturation_limit -> Limite di saturazione (valore assoluto)
    %
    % OUTPUT:
    % V_d_ref         -> Uscita del controllore PI con saturazione
    
    % Definizione di variabili statiche per la memoria interna del PI
    persistent integrator_state;
    if isempty(integrator_state)
        integrator_state = single(0);  % Inizializza la memoria dell'integratore
    end
    
    % Reset integratore se richiesto
    if reset
        integrator_state = Id0;
    end
    
    % Parte proporzionale
    P_term = P * e;
    
    % Parte integrale (accumulatore)
    integrator_state = integrator_state + I_Ts_speed * e;
    
    % Uscita PI senza saturazione
    V_d_ref_unsat = P_term + integrator_state;
    
    % Saturazione dell'uscita (limite superiore e inferiore)
    V_d_ref = max(min(V_d_ref_unsat, saturation_limit), -saturation_limit);
    
    % Implementazione dell'anti-windup: corregge l'integratore in caso di saturazione
    if V_d_ref ~= V_d_ref_unsat
        integrator_state = integrator_state - I_Ts_speed * e;  % Evita windup
    end
end

== matlab function mcb_pmsm_foc_f28379d_dyno/Current control for motor1/Control_System/Closed Loop Control/Current_Controllers/PI_Controller_Iq/MATLAB Function ==
  data: e input; V_q_ref output; P input; I_Ts_speed input; reset input; Iq0 input; saturation_limit input
function V_q_ref = PI_Controller(e, P, I_Ts_speed, reset, Iq0, saturation_limit)
    % PI_Controller: implementa un controllore PI con saturazione e reset.
    % INPUTS:
    % e               -> Errore (input del PI)
    % P               -> Guadagno proporzionale
    % I_Ts_speed      -> Guadagno integrale moltiplicato per Ts (I*Ts_speed)
    % reset           -> Segnale booleano per resettare l'integratore
    % Iq0              -> Valore iniziale del riferimento (per l'integratore)
    % saturation_limit -> Limite di saturazione (valore assoluto)
    %
    % OUTPUT:
    % V_q_ref         -> Uscita del controllore PI con saturazione
    
    % Definizione di variabili statiche per la memoria interna del PI
    persistent integrator_state;
    if isempty(integrator_state)
        integrator_state = single(0);  % Inizializza la memoria dell'integratore
    end
    
    % Reset integratore se richiesto
    if reset
        integrator_state = Iq0;
    end
    
    % Parte proporzionale
    P_term = P * e;
    
    % Parte integrale (accumulatore)
    integrator_state = integrator_state + I_Ts_speed * e;
    
    % Uscita PI senza saturazione
    V_q_ref_unsat = P_term + integrator_state;
    
    % Saturazione dell'uscita (limite superiore e inferiore)
    V_q_ref = max(min(V_q_ref_unsat, saturation_limit), -saturation_limit);
    
    % Implementazione dell'anti-windup: corregge l'integratore in caso di saturazione
    if V_q_ref ~= V_q_ref_unsat
        integrator_state = integrator_state - I_Ts_speed * e;  % Evita windup
    end
end

== matlab function mcb_pmsm_foc_f28379d_dyno/Current control for motor2/Control_System/Closed Loop Control/Current_Controllers/PI_Controller_Iq/MATLAB Function ==
  data: e input; V_q_ref output; P input; I_Ts_speed input; reset input; Iq0 input; saturation_limit input
function V_q_ref = PI_Controller(e, P, I_Ts_speed, reset, Iq0, saturation_limit)
    % PI_Controller: implementa un controllore PI con saturazione e reset.
    % INPUTS:
    % e               -> Errore (input del PI)
    % P               -> Guadagno proporzionale
    % I_Ts_speed      -> Guadagno integrale moltiplicato per Ts (I*Ts_speed)
    % reset           -> Segnale booleano per resettare l'integratore
    % Iq0              -> Valore iniziale del riferimento (per l'integratore)
    % saturation_limit -> Limite di saturazione (valore assoluto)
    %
    % OUTPUT:
    % V_q_ref         -> Uscita del controllore PI con saturazione
    
    % Definizione di variabili statiche per la memoria interna del PI
    persistent integrator_state;
    if isempty(integrator_state)
        integrator_state = single(0);  % Inizializza la memoria dell'integratore
    end
    
    % Reset integratore se richiesto
    if reset
        integrator_state = Iq0;
    end
    
    % Parte proporzionale
    P_term = P * e;
    
    % Parte integrale (accumulatore)
    integrator_state = integrator_state + I_Ts_speed * e;
    
    % Uscita PI senza saturazione
    V_q_ref_unsat = P_term + integrator_state;
    
    % Saturazione dell'uscita (limite superiore e inferiore)
    V_q_ref = max(min(V_q_ref_unsat, saturation_limit), -saturation_limit);
    
    % Implementazione dell'anti-windup: corregge l'integratore in caso di saturazione
    if V_q_ref ~= V_q_ref_unsat
        integrator_state = integrator_state - I_Ts_speed * e;  % Evita windup
    end
end

== matlab function mcb_pmsm_foc_f28379d_dyno/Speed control for motor1/PI_Controller_Speed/MATLAB Function1 ==
  data: error input; ISE output; Ts input; IAE output; ITAE output
function [ISE,IAE,ITAE] = computeIndices(error, Ts)
    persistent t;
    persistent old_index;

    if isempty(t)
        t=single(0);
    end
    if isempty(old_index)
        old_index.ISE = single(0);
        old_index.IAE = single(0);
        old_index.ITAE = single(0);
    end
    ISE = old_index.ISE + (error^2) * Ts;
    IAE = old_index.IAE + abs(error) * Ts;
    ITAE = old_index.ITAE + t * abs(error) * Ts;
    disp(t)
    if t>=10
        assignin('base', 'ISE', ISE);
        assignin('base', 'IAE', IAE);
        assignin('base', 'ITAE', ITAE);
    else
        t=t+Ts;
        old_index.ISE=ISE;
        old_index.IAE=IAE;
        old_index.ITAE=ITAE;
    end
end
